simulink library "GTM_aerolib"  (R2023b)
settings: Solver=ode45  StartTime=0.0  StopTime=10.0  RelTol=1e-3
undefined symbols (not defined in the file or in its folder): Aero, DamageModels
libraries: simulink_need_slupdate x58, $bdroot x4, simulink x3
(part 1 of 2)
settings Model: Creator=cox  LastModifiedBy=suvo
settings SolverCC: AlgebraicLoopSolver=TrustRegion
settings DataIOCC: LimitDataPoints=on  SaveFormat=Array  SignalLoggingSaveFormat=ModelDataLogs  ReturnWorkspaceOutputs=off
settings OptimizationCC: BlockReduction=off  BooleanDataType=off  ExpressionDepthLimit=2147483647  LifeSpan=inf
settings DebuggingCC: SaveWithParameterizedLinksMsg=none  UnderspecifiedInitializationDetection=Classic  MergeDetectMultiDrivingBlocksExec=none  SignalResolutionControl=TryResolveAllWithWarning  FcnCallInpInsideContextMsg=warning  UnconnectedInputMsg=warning  UnconnectedOutputMsg=warning  UnconnectedLineMsg=warning  StateNameClashWarn=warning  SFUnexpectedBacktrackingDiag=warning  SFNoUnconditionalDefaultTransitionDiag=warning  SFExecutionAtInitializationDiag=none  ArithmeticOperatorsInVariantConditions=warning
settings HardwareCC: ProdBitPerPointer=32  ProdBitPerSizeT=32  ProdBitPerPtrDiffT=32  ProdLargestAtomicFloat=None  ProdIntDivRoundTo=Undefined  ProdEndianess=Unspecified  ProdWordSize=32  ProdHWDeviceType=32-bit Generic  TargetUnknown=on
settings ModelReferenceCC: PropagateSignalLabelsOutOfModel=off
settings SFSimCC: SimUseLocalCustomCode=off  CustomCodeUndefinedFunction=UseInterfaceOnly
settings RTWCC: RTWUseLocalCustomCode=off
settings CodeAppCC: StateflowObjectComments=on
settings GRTTargetCC: TargetLangStandard=C89/C90 (ANSI)  CombineOutputUpdateFcns=off  GRTInterface=on
settings ConfigComp: CovMetricSettings=dw  CovSaveCumulativeToWorkspaceVar=on  CovSaveSingleToWorkspaceVar=on

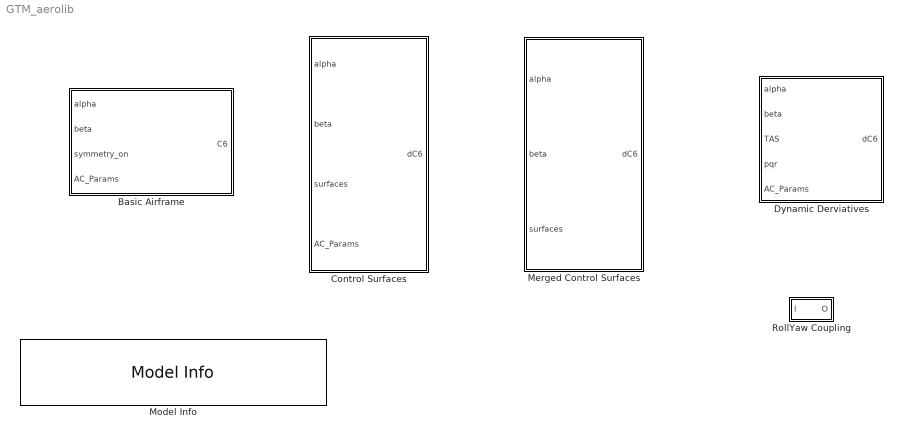
== system GTM_aerolib ==
  Basic Airframe : Subsystem
  Control Surfaces : Subsystem
  Dynamic Derviatives : Subsystem
  Merged Control Surfaces : Subsystem
  Model Info : simulink/Model-Wide Utilities/Model Info  Frame=on  DisplayStringWithTags=|  HorizontalTextAlignment=Center  LeftAlignmentValue=0.5
      | GTM AeroTables
      | Subversion Info: %<ModelVersion>
      | Last modified by %<LastModifiedBy> on %<LastModificationDate>
  RollYaw Coupling : Subsystem  mask{arm=-0.07}
      mask prompts: arm "Moment arm (nd)"
      mask help:
      | Approximates roll/yaw coupling of split longitudinal surface
      | deflections (spoilers, elevators, flaps) where the base aero data only
      | has CX, CZ, and Cm. Input should be a 6 element vector of the aero
      | coefficients [CZ CY CZ Cl Cm Cn].
      |
      | Cl = Cl_input + arm*CZ_input
      | Cn = Cn_input + arm*CX_input
      mask init:
      | Kc = eye(6);
      | 
      | Kc(4,3) = arm; % Cl = Cl + arm*CZ
      | Kc(6,1) = arm; % Cn = Cn + arm*CX

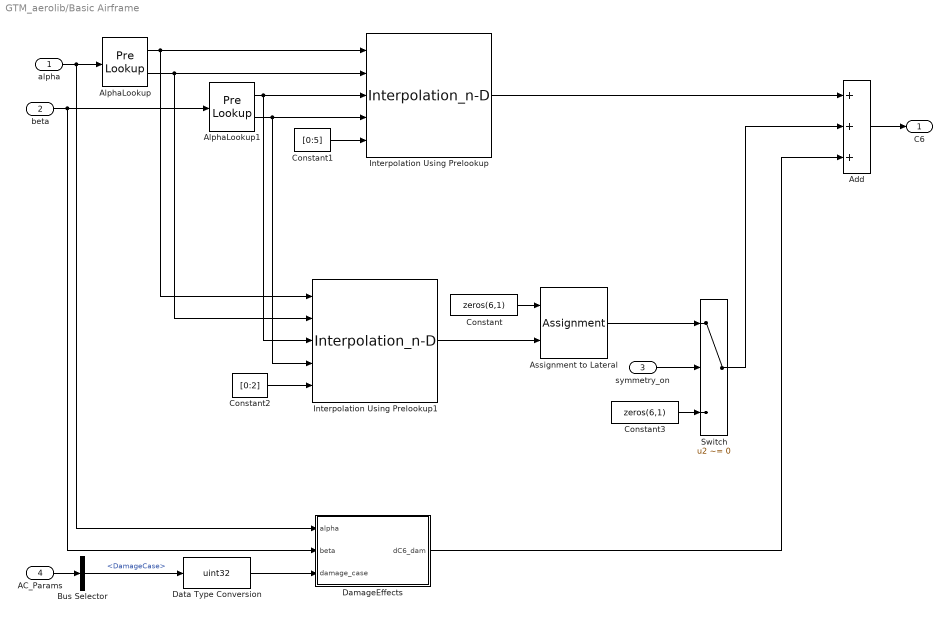
== system GTM_aerolib/Basic Airframe ==
  alpha : Inport
  beta : Inport  Port=2
  symmetry_on : Inport  Port=3
  AC_Params : Inport  Port=4
  Add : Sum  Inputs=+++
  AlphaLookup : PreLookup  BreakpointsData=Aero.C6_bas.alpha  IndexSearchMethod=Linear search  BeginIndexSearchUsingPreviousIndexResult=on  ExtrapMethod=Linear
  AlphaLookup1 : PreLookup  BreakpointsData=Aero.C6_bas.beta  IndexSearchMethod=Linear search  BeginIndexSearchUsingPreviousIndexResult=on  ExtrapMethod=Linear
  Assignment to Lateral : Assignment  IndexMode=Zero-based  IndexOptions=Index vector (dialog)  Indices=[1 3 5]  OutputSizes=[1 1]
  Bus Selector : BusSelector  OutputSignals=DamageCase
  Constant : Constant  Value=zeros(6,1)
  Constant1 : Constant  Value=[0:5]  OutDataTypeStr=uint32
  Constant2 : Constant  Value=[0:2]  OutDataTypeStr=uint32
  Constant3 : Constant  Value=zeros(6,1)
  DamageEffects : Subsystem
  Data Type Conversion : DataTypeConversion  OutDataTypeStr=uint32  RndMeth=Nearest  SaturateOnIntegerOverflow=off
  Interpolation Using Prelookup : Interpolation_n-D  NumberOfTableDimensions=3  Table=Aero.C6_bas.data  NumSelectionDims=1
      settings: InputPortMap=u0,u1,u2,u3,u4
  Interpolation Using Prelookup1 : Interpolation_n-D  NumberOfTableDimensions=3  Table=Aero.dC3_sym.data  NumSelectionDims=1
      settings: InputPortMap=u0,u1,u2,u3,u4
  Switch : Switch  Criteria=u2 ~= 0  SaturateOnIntegerOverflow=off  InputSameDT=off
  C6 : Outport
  wires:
  Interpolation Using Prelookup/1 -> Add/1
  Constant/1 -> Assignment to Lateral/1
  Interpolation Using Prelookup1/1 -> Assignment to Lateral/2
  Constant3/1 -> Switch/3
  Assignment to Lateral/1 -> Switch/1
  symmetry_on/1 -> Switch/2
  Add/1 -> C6/1
  Switch/1 -> Add/2
  alpha/1 -> DamageEffects/1(alpha), AlphaLookup/1
  beta/1 -> DamageEffects/2(beta), AlphaLookup1/1
  DamageEffects/1(dC6_dam) -> Add/3
  AC_Params/1 -> Bus Selector/1
  Bus Selector/1 -> Data Type Conversion/1  "<DamageCase>"
  AlphaLookup/1 -> Interpolation Using Prelookup/1, Interpolation Using Prelookup1/1
  AlphaLookup/2 -> Interpolation Using Prelookup/2, Interpolation Using Prelookup1/2
  AlphaLookup1/1 -> Interpolation Using Prelookup/3, Interpolation Using Prelookup1/3
  AlphaLookup1/2 -> Interpolation Using Prelookup/4, Interpolation Using Prelookup1/4
  Constant1/1 -> Interpolation Using Prelookup/5
  Constant2/1 -> Interpolation Using Prelookup1/5
  Data Type Conversion/1 -> DamageEffects/3(damage_case)

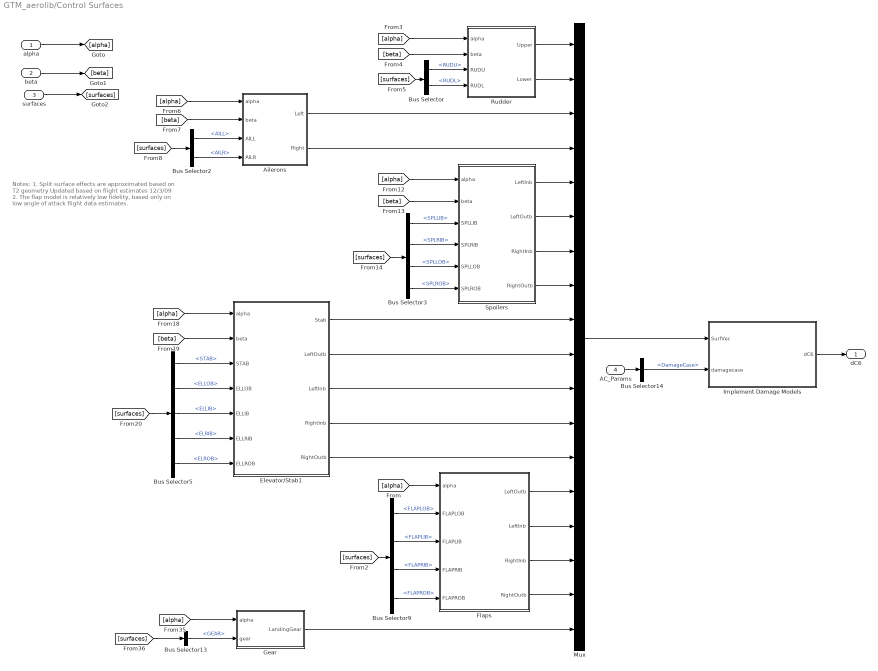
== system GTM_aerolib/Control Surfaces ==
  note: Notes:
      | 1. Split surface effects are approximated
      | based on T2 geometry
      | Updated based on flight estimates 12/3/09
      |
      | 2. The flap model is relatively low fidelity, based
      | only on low angle of attack flight data estimates.
  alpha : Inport
  beta : Inport  Port=2  PortDimensions=1
  surfaces : Inport  Port=3
  AC_Params : Inport  Port=4
  Ailerons : Subsystem
  Bus Selector : BusSelector  OutputSignals=RUDU,RUDL
  Bus Selector13 : BusSelector  OutputSignals=GEAR
  Bus Selector14 : BusSelector  OutputSignals=DamageCase
  Bus Selector2 : BusSelector  OutputSignals=AILL,AILR
  Bus Selector3 : BusSelector  OutputSignals=SPLLIB,SPLRIB,SPLLOB,SPLROB
  Bus Selector5 : BusSelector  OutputSignals=STAB,ELLOB,ELLIB,ELRIB,ELROB
  Bus Selector9 : BusSelector  OutputSignals=FLAPLOB,FLAPLIB,FLAPRIB,FLAPROB
  Elevator/Stab1 : Subsystem
  Flaps : Subsystem
  Gear : Subsystem
  Implement Damage Models : Subsystem  mask{DamageModels=DamageModels}
      mask prompts: DamageModels "Cell Array of Damage Models"
      mask help: Implements Damage Models as gain and bias effects on selected surfaces.
      mask init:
      | SurfList={...
      |     'RUDU','RUDL',...
      |     'AILL','AILR',...
      |     'SPLLIB','SPLRIB','SPLLOB','SPLROB',...
      |     'STAB',...
      |     'ELLOB','ELLIB','ELRIB','ELROB',...
      |     'FLAPLOB','FALPLIB','FLAPRIB','FLAPROB',...
      |     'GEAR'
      |     };
      | 
      | Ncases=length(DamageModels);
      | Nsurfs=length(SurfList);
      | SurfGain=ones(Ncases,Nsurfs,6);   %Nominally unity gain, zero bias
      | 
      | %If damage case includes gain/bias on a surface adjust nominal values
      | % First damage case is "no damage".
      | for i=1:Ncases,
      |  for j=1:Nsurfs,
      |     if isfield(DamageModels{i},SurfList{j}),
      |         SurfGain(i,j,:)=DamageModels{i}.(SurfList{j}).gain*ones(1,6);
      |     end
      |  end
      | end
  Mux : Mux  Inputs=18
  Rudder : Subsystem
  Spoilers : Subsystem
  dC6 : Outport
  wires:
  Bus Selector13/1 -> Gear/2(gear)  "<GEAR>"
  [alpha] -> Gear/1(alpha)
  [surfaces] -> Bus Selector13/1
  [alpha] -> Flaps/1(alpha)
  [surfaces] -> Bus Selector9/1
  Bus Selector5/2 -> Elevator/Stab1/4(ELLOB)  "<ELLOB>"
  Bus Selector5/1 -> Elevator/Stab1/3(STAB)  "<STAB>"
  [alpha] -> Elevator/Stab1/1(alpha)
  [surfaces] -> Bus Selector5/1
  [beta] -> Elevator/Stab1/2(beta)
  Bus Selector3/2 -> Spoilers/4(SPLRIB)  "<SPLRIB>"
  Bus Selector3/1 -> Spoilers/3(SPLLIB)  "<SPLLIB>"
  [surfaces] -> Bus Selector3/1
  [beta] -> Spoilers/2(beta)
  [alpha] -> Spoilers/1(alpha)
  Bus Selector2/2 -> Ailerons/4(AILR)  "<AILR>"
  Bus Selector2/1 -> Ailerons/3(AILL)  "<AILL>"
  [surfaces] -> Bus Selector2/1
  [beta] -> Ailerons/2(beta)
  [alpha] -> Ailerons/1(alpha)
  Bus Selector/2 -> Rudder/4(RUDL)  "<RUDL>"
  Bus Selector/1 -> Rudder/3(RUDU)  "<RUDU>"
  [surfaces] -> Bus Selector/1
  [beta] -> Rudder/2(beta)
  [alpha] -> Rudder/1(alpha)
  surfaces/1 -> [surfaces]
  beta/1 -> [beta]
  alpha/1 -> [alpha]
  AC_Params/1 -> Bus Selector14/1
  Bus Selector3/3 -> Spoilers/5(SPLLOB)  "<SPLLOB>"
  Bus Selector3/4 -> Spoilers/6(SPLROB)  "<SPLROB>"
  Bus Selector5/3 -> Elevator/Stab1/5(ELLIB)  "<ELLIB>"
  Bus Selector5/4 -> Elevator/Stab1/6(ELLRIB)  "<ELRIB>"
  Bus Selector5/5 -> Elevator/Stab1/7(ELLROB)  "<ELROB>"
  Rudder/1(Upper) -> Mux/1
  Rudder/2(Lower) -> Mux/2
  Ailerons/1(Left) -> Mux/3
  Ailerons/2(Right) -> Mux/4
  Spoilers/1(LeftInb) -> Mux/5
  Spoilers/2(LeftOutb) -> Mux/6
  Spoilers/3(RightInb) -> Mux/7
  Spoilers/4(RightOutb) -> Mux/8
  Elevator/Stab1/1(Stab) -> Mux/9
  Elevator/Stab1/2(LeftOutb) -> Mux/10
  Elevator/Stab1/3(LeftInb) -> Mux/11
  Elevator/Stab1/4(RightInb) -> Mux/12
  Elevator/Stab1/5(RightOutb) -> Mux/13
  Gear/1(LandingGear) -> Mux/18
  Flaps/1(LeftOutb) -> Mux/14
  Flaps/2(LeftInb) -> Mux/15
  Flaps/3(RightInb) -> Mux/16
  Flaps/4(RightOutb) -> Mux/17
  Bus Selector14/1 -> Implement Damage Models/2(damagecase)  "<DamageCase>"
  Mux/1 -> Implement Damage Models/1(SurfVec)
  Implement Damage Models/1(dC6) -> dC6/1
  Bus Selector9/1 -> Flaps/2(FLAPLOB)  "<FLAPLOB>"
  Bus Selector9/2 -> Flaps/3(FLAPLIB)  "<FLAPLIB>"
  Bus Selector9/3 -> Flaps/4(FLAPRIB)  "<FLAPRIB>"
  Bus Selector9/4 -> Flaps/5(FLAPROB)  "<FLAPROB>"

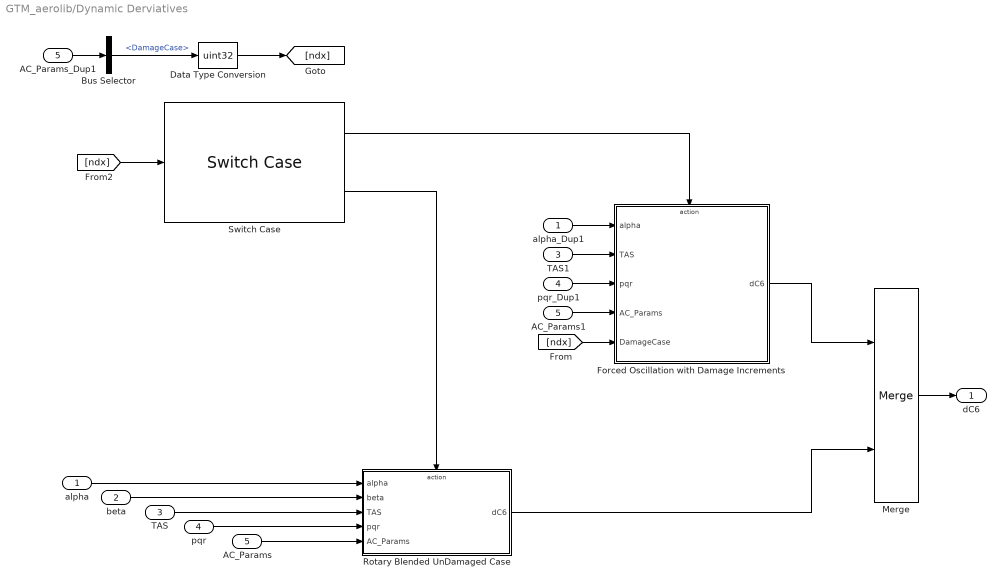
== system GTM_aerolib/Dynamic Derviatives ==
  alpha : Inport
  beta : Inport  Port=2
  TAS : Inport  Port=3
  pqr : Inport  Port=4
  AC_Params : Inport  Port=5
  AC_Params1 : InportShadow  Port=5
  AC_Params_Dup1 : InportShadow  Port=5
  Bus Selector : BusSelector  OutputSignals=DamageCase
  Data Type Conversion : DataTypeConversion  OutDataTypeStr=uint32  RndMeth=Nearest  SaturateOnIntegerOverflow=off
  Forced Oscillation with Damage Increments : Subsystem
  Merge : Merge  InitialOutput=zeros(6,1)
  Rotary Blended UnDamaged Case : Subsystem
  Switch Case : SwitchCase  CaseConditions={[1,2,3,4,5,6]}
  TAS1 : InportShadow  Port=3
  alpha_Dup1 : InportShadow
  pqr_Dup1 : InportShadow  Port=4
  dC6 : Outport
  wires:
  alpha/1 -> Rotary Blended UnDamaged Case/1(alpha)
  beta/1 -> Rotary Blended UnDamaged Case/2(beta)
  TAS/1 -> Rotary Blended UnDamaged Case/3(TAS)
  pqr/1 -> Rotary Blended UnDamaged Case/4(pqr)
  AC_Params/1 -> Rotary Blended UnDamaged Case/5(AC_Params)
  Merge/1 -> dC6/1
  Switch Case/1 -> Forced Oscillation with Damage Increments/Action
  Switch Case/2 -> Rotary Blended UnDamaged Case/Action
  Rotary Blended UnDamaged Case/1(dC6) -> Merge/2
  Bus Selector/1 -> Data Type Conversion/1  "<DamageCase>"
  AC_Params_Dup1/1 -> Bus Selector/1
  Data Type Conversion/1 -> [ndx]
  [ndx] -> Switch Case/1
  alpha_Dup1/1 -> Forced Oscillation with Damage Increments/1(alpha)
  TAS1/1 -> Forced Oscillation with Damage Increments/2(TAS)
  pqr_Dup1/1 -> Forced Oscillation with Damage Increments/3(pqr)
  AC_Params1/1 -> Forced Oscillation with Damage Increments/4(AC_Params)
  [ndx] -> Forced Oscillation with Damage Increments/5(DamageCase)
  Forced Oscillation with Damage Increments/1(dC6) -> Merge/1

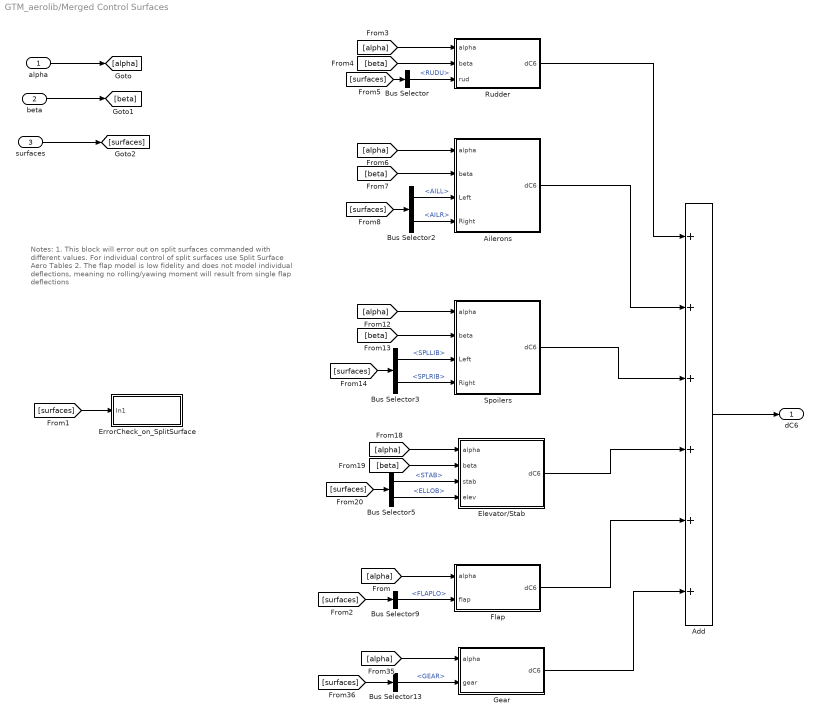
== system GTM_aerolib/Merged Control Surfaces ==
  note: Notes:
      | 1. This block will error out on split surfaces commanded
      | with different values.  For individual control of split surfaces
      | use Split Surface Aero Tables
      |
      | 2. The flap model is low fidelity and does
      | not model individual deflections, meaning
      | no rolling/yawing moment will result
      | from single flap deflections
  alpha : Inport
  beta : Inport  Port=2  PortDimensions=1
  surfaces : Inport  Port=3
  Add : Sum  Inputs=++++++
  Ailerons : Subsystem
  Bus Selector : BusSelector  OutputSignals=RUDU
  Bus Selector13 : BusSelector  OutputSignals=GEAR
  Bus Selector2 : BusSelector  OutputSignals=AILL,AILR
  Bus Selector3 : BusSelector  OutputSignals=SPLLIB,SPLRIB
  Bus Selector5 : BusSelector  OutputSignals=STAB,ELLOB
  Bus Selector9 : BusSelector  OutputSignals=FLAPLO
  Elevator/Stab : Subsystem
  ErrorCheck_on_SplitSurface : Subsystem
  Flap : Subsystem
  Gear : Subsystem
  Rudder : Subsystem
  Spoilers : Subsystem
  dC6 : Outport
  wires:
  Add/1 -> dC6/1
  alpha/1 -> [alpha]
  beta/1 -> [beta]
  surfaces/1 -> [surfaces]
  [alpha] -> Rudder/1(alpha)
  [beta] -> Rudder/2(beta)
  [surfaces] -> Bus Selector/1
  Bus Selector/1 -> Rudder/3(rud)  "<RUDU>"
  [alpha] -> Ailerons/1(alpha)
  [beta] -> Ailerons/2(beta)
  [surfaces] -> Bus Selector2/1
  Bus Selector2/1 -> Ailerons/3(Left)  "<AILL>"
  Bus Selector2/2 -> Ailerons/4(Right)  "<AILR>"
  [alpha] -> Spoilers/1(alpha)
  [beta] -> Spoilers/2(beta)
  [surfaces] -> Bus Selector3/1
  Bus Selector3/1 -> Spoilers/3(Left)  "<SPLLIB>"
  Bus Selector3/2 -> Spoilers/4(Right)  "<SPLRIB>"
  [beta] -> Elevator/Stab/2(beta)
  [surfaces] -> Bus Selector5/1
  [alpha] -> Elevator/Stab/1(alpha)
  Bus Selector5/1 -> Elevator/Stab/3(stab)  "<STAB>"
  Bus Selector5/2 -> Elevator/Stab/4(elev)  "<ELLOB>"
  [surfaces] -> Bus Selector9/1
  [alpha] -> Flap/1(alpha)
  Bus Selector9/1 -> Flap/2(flap)  "<FLAPLO>"
  [surfaces] -> Bus Selector13/1
  [alpha] -> Gear/1(alpha)
  Bus Selector13/1 -> Gear/2(gear)  "<GEAR>"
  Rudder/1(dC6) -> Add/1
  Ailerons/1(dC6) -> Add/2
  Spoilers/1(dC6) -> Add/3
  Elevator/Stab/1(dC6) -> Add/4
  Flap/1(dC6) -> Add/5
  Gear/1(dC6) -> Add/6
  [surfaces] -> ErrorCheck_on_SplitSurface/1(In1)

== system GTM_aerolib/RollYaw Coupling ==
  I : Inport
  Gain : Gain  Gain=Kc  Multiplication=Matrix(K*u)
  O : Outport
  wires:
  I/1 -> Gain/1
  Gain/1 -> O/1

== system GTM_aerolib/Basic Airframe/DamageEffects ==
  alpha : Inport
  beta : Inport  Port=2
  damage_case : Inport  Port=3
  Merge : Merge  InitialOutput=zeros(6,1)
  Switch Case : SwitchCase  CaseConditions={[1,2,3,4,5,6]}
  Switch Case Action Subsystem : Subsystem  TreatAsAtomicUnit=on
  Switch Case Action Subsystem2 : Subsystem  TreatAsAtomicUnit=on
  damage_case_DUP : InportShadow  Port=3
  dC6_dam : Outport
  wires:
  Switch Case/2 -> Switch Case Action Subsystem2/Action
  Switch Case Action Subsystem2/1(Zeros) -> Merge/2
  alpha/1 -> Switch Case Action Subsystem/1(alpha)
  beta/1 -> Switch Case Action Subsystem/2(beta)
  Merge/1 -> dC6_dam/1
  damage_case/1 -> Switch Case/1
  Switch Case/1 -> Switch Case Action Subsystem/Action
  Switch Case Action Subsystem/1(dC6_dam) -> Merge/1
  damage_case_DUP/1 -> Switch Case Action Subsystem/3(damage_case)

== system GTM_aerolib/Control Surfaces/Ailerons ==
  alpha : Inport
  beta : Inport  Port=2
  AILL : Inport  Port=3
  AILR : Inport  Port=4
  Constant1 : Constant  Value=[0:5]  OutDataTypeStr=uint32
  Constant3 : Constant  Value=[0:5]  OutDataTypeStr=uint32
  Gain2 : Gain  Gain=-1
  Interpolation Using Prelookup : Interpolation_n-D  NumberOfTableDimensions=4  Table=Aero.dC6_ail.data  NumSelectionDims=1
      settings: InputPortMap=u0,u1,u2,u3,u4,u5,u6
  Interpolation Using Prelookup1 : Interpolation_n-D  NumberOfTableDimensions=4  Table=Aero.dC6_ail.data  NumSelectionDims=1
      settings: InputPortMap=u0,u1,u2,u3,u4,u5,u6
  Negate Lateral : Gain  Gain=[1 -1 1 -1 1 -1]
  Prelookup1 : PreLookup  BreakpointsData=Aero.dC6_ail.alpha  IndexSearchMethod=Linear search  BeginIndexSearchUsingPreviousIndexResult=on  ExtrapMethod=Linear
  Prelookup2 : PreLookup  BreakpointsData=Aero.dC6_ail.beta  IndexSearchMethod=Linear search  BeginIndexSearchUsingPreviousIndexResult=on  ExtrapMethod=Linear
  Prelookup3 : PreLookup  BreakpointsData=Aero.dC6_ail.ail  IndexSearchMethod=Linear search  BeginIndexSearchUsingPreviousIndexResult=on  ExtrapMethod=Linear
  Prelookup4 : PreLookup  BreakpointsData=Aero.dC6_ail.beta  IndexSearchMethod=Linear search  BeginIndexSearchUsingPreviousIndexResult=on  ExtrapMethod=Linear
  Prelookup5 : PreLookup  BreakpointsData=Aero.dC6_ail.ail  IndexSearchMethod=Linear search  BeginIndexSearchUsingPreviousIndexResult=on  ExtrapMethod=Linear
  Left : Outport
  Right : Outport  Port=2
  wires:
  Gain2/1 -> Prelookup2/1
  Negate Lateral/1 -> Left/1
  Interpolation Using Prelookup1/1 -> Right/1
  AILR/1 -> Prelookup5/1
  beta/1 -> Gain2/1, Prelookup4/1
  alpha/1 -> Prelookup1/1
  AILL/1 -> Prelookup3/1
  Prelookup1/1 -> Interpolation Using Prelookup/1, Interpolation Using Prelookup1/1
  Prelookup1/2 -> Interpolation Using Prelookup/2, Interpolation Using Prelookup1/2
  Prelookup2/1 -> Interpolation Using Prelookup/3
  Prelookup2/2 -> Interpolation Using Prelookup/4
  Prelookup3/1 -> Interpolation Using Prelookup/5
  Prelookup3/2 -> Interpolation Using Prelookup/6
  Constant3/1 -> Interpolation Using Prelookup/7
  Prelookup4/1 -> Interpolation Using Prelookup1/3
  Prelookup4/2 -> Interpolation Using Prelookup1/4
  Prelookup5/1 -> Interpolation Using Prelookup1/5
  Prelookup5/2 -> Interpolation Using Prelookup1/6
  Constant1/1 -> Interpolation Using Prelookup1/7
  Interpolation Using Prelookup/1 -> Negate Lateral/1

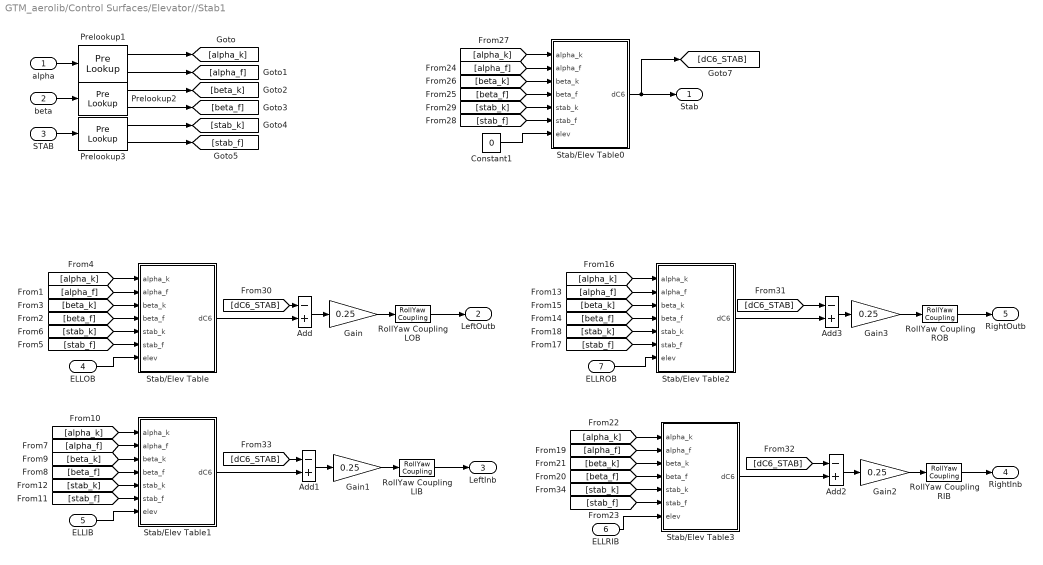
== system GTM_aerolib/Control Surfaces/Elevator//Stab1 ==
  alpha : Inport
  beta : Inport  Port=2
  STAB : Inport  Port=3
  ELLOB : Inport  Port=4
  ELLIB : Inport  Port=5
  ELLRIB : Inport  Port=6
  ELLROB : Inport  Port=7
  Add{,1..3} (4 alike) : Sum  Inputs=-+
  Constant1 : Constant  Value=0
  Gain{,1..3} (4 alike) : Gain  Gain=0.25
  Prelookup1 : PreLookup  BreakpointsData=Aero.dC3_ele.alpha  IndexSearchMethod=Linear search  BeginIndexSearchUsingPreviousIndexResult=on  ExtrapMethod=Linear
  Prelookup2 : PreLookup  BreakpointsData=Aero.dC3_ele.beta  IndexSearchMethod=Linear search  BeginIndexSearchUsingPreviousIndexResult=on  ExtrapMethod=Linear
  Prelookup3 : PreLookup  BreakpointsData=Aero.dC3_ele.stab  IndexSearchMethod=Linear search  BeginIndexSearchUsingPreviousIndexResult=on  ExtrapMethod=Linear
  RollYaw Coupling LIB : $bdroot/RollYaw Coupling  SystemSampleTime=-1  arm=-0.03
  RollYaw Coupling LOB : $bdroot/RollYaw Coupling  SystemSampleTime=-1  arm=-0.07
  RollYaw Coupling RIB : $bdroot/RollYaw Coupling  SystemSampleTime=-1  arm=0.03
  RollYaw Coupling ROB : $bdroot/RollYaw Coupling  SystemSampleTime=-1  arm=0.07
  Stab/Elev Table : Subsystem
  Stab/Elev Table0 : Subsystem
  Stab/Elev Table1 : Subsystem
  Stab/Elev Table2 : Subsystem
  Stab/Elev Table3 : Subsystem
  Stab : Outport
  LeftOutb : Outport  Port=2
  LeftInb : Outport  Port=3
  RightInb : Outport  Port=4
  RightOutb : Outport  Port=5
  wires:
  alpha/1 -> Prelookup1/1
  beta/1 -> Prelookup2/1
  STAB/1 -> Prelookup3/1
  Prelookup1/1 -> [alpha_k]
  Prelookup1/2 -> [alpha_f]
  Prelookup2/1 -> [beta_k]
  Prelookup2/2 -> [beta_f]
  Prelookup3/1 -> [stab_k]
  Prelookup3/2 -> [stab_f]
  Gain/1 -> RollYaw Coupling LOB/1
  Gain1/1 -> RollYaw Coupling LIB/1
  Gain2/1 -> RollYaw Coupling RIB/1
  Gain3/1 -> RollYaw Coupling ROB/1
  Add/1 -> Gain/1
  Add1/1 -> Gain1/1
  Add2/1 -> Gain2/1
  Add3/1 -> Gain3/1
  [alpha_k] -> Stab/Elev Table/1(alpha_k)
  [alpha_f] -> Stab/Elev Table/2(alpha_f)
  [beta_k] -> Stab/Elev Table/3(beta_k)
  [beta_f] -> Stab/Elev Table/4(beta_f)
  [stab_k] -> Stab/Elev Table/5(stab_k)
  [stab_f] -> Stab/Elev Table/6(stab_f)
  ELLOB/1 -> Stab/Elev Table/7(elev)
  [alpha_k] -> Stab/Elev Table1/1(alpha_k)
  [alpha_f] -> Stab/Elev Table1/2(alpha_f)
  [beta_k] -> Stab/Elev Table1/3(beta_k)
  [beta_f] -> Stab/Elev Table1/4(beta_f)
  [stab_k] -> Stab/Elev Table1/5(stab_k)
  [stab_f] -> Stab/Elev Table1/6(stab_f)
  ELLIB/1 -> Stab/Elev Table1/7(elev)
  [alpha_k] -> Stab/Elev Table2/1(alpha_k)
  [alpha_f] -> Stab/Elev Table2/2(alpha_f)
  [beta_k] -> Stab/Elev Table2/3(beta_k)
  [beta_f] -> Stab/Elev Table2/4(beta_f)
  [stab_k] -> Stab/Elev Table2/5(stab_k)
  [stab_f] -> Stab/Elev Table2/6(stab_f)
  ELLROB/1 -> Stab/Elev Table2/7(elev)
  [alpha_k] -> Stab/Elev Table3/1(alpha_k)
  [alpha_f] -> Stab/Elev Table3/2(alpha_f)
  [beta_k] -> Stab/Elev Table3/3(beta_k)
  [beta_f] -> Stab/Elev Table3/4(beta_f)
  [stab_k] -> Stab/Elev Table3/5(stab_k)
  [stab_f] -> Stab/Elev Table3/6(stab_f)
  ELLRIB/1 -> Stab/Elev Table3/7(elev)
  Stab/Elev Table/1(dC6) -> Add/2
  [dC6_STAB] -> Add/1
  [alpha_k] -> Stab/Elev Table0/1(alpha_k)
  [alpha_f] -> Stab/Elev Table0/2(alpha_f)
  [beta_k] -> Stab/Elev Table0/3(beta_k)
  [beta_f] -> Stab/Elev Table0/4(beta_f)
  [stab_k] -> Stab/Elev Table0/5(stab_k)
  [stab_f] -> Stab/Elev Table0/6(stab_f)
  Constant1/1 -> Stab/Elev Table0/7(elev)
  Stab/Elev Table1/1(dC6) -> Add1/2
  Stab/Elev Table2/1(dC6) -> Add3/2
  [dC6_STAB] -> Add3/1
  [dC6_STAB] -> Add2/1
  Stab/Elev Table3/1(dC6) -> Add2/2
  [dC6_STAB] -> Add1/1
  Stab/Elev Table0/1(dC6) -> Stab/1, [dC6_STAB]
  RollYaw Coupling LOB/1 -> LeftOutb/1
  RollYaw Coupling LIB/1 -> LeftInb/1
  RollYaw Coupling ROB/1 -> RightOutb/1
  RollYaw Coupling RIB/1 -> RightInb/1

== system GTM_aerolib/Control Surfaces/Flaps ==
  alpha : Inport
  FLAPLOB : Inport  Port=2
  FLAPLIB : Inport  Port=3
  FLAPRIB : Inport  Port=4
  FLAPROB : Inport  Port=5
  Gain : Gain  Gain=Aero.flaps.flaplob
  Gain1 : Gain  Gain=Aero.flaps.flaplib
  Gain2 : Gain  Gain=Aero.flaps.flaprib
  Gain3 : Gain  Gain=Aero.flaps.flaprob
  Terminator : Terminator
  LeftOutb : Outport
  LeftInb : Outport  Port=2
  RightInb : Outport  Port=3
  RightOutb : Outport  Port=4
  wires:
  alpha/1 -> Terminator/1
  FLAPLOB/1 -> Gain/1
  FLAPLIB/1 -> Gain1/1
  FLAPRIB/1 -> Gain2/1
  FLAPROB/1 -> Gain3/1
  Gain/1 -> LeftOutb/1
  Gain1/1 -> LeftInb/1
  Gain2/1 -> RightInb/1
  Gain3/1 -> RightOutb/1

== system GTM_aerolib/Control Surfaces/Gear ==
  alpha : Inport
  gear : Inport  Port=2
  Assignment to Longitudinal : Assignment  IndexMode=Zero-based  IndexOptions=Index vector (dialog)  Indices=[0 2 4]  OutputSizes=[1 1]
  Compare To Zero : simulink/Logic and Bit Operations/Compare To Zero  SystemSampleTime=-1  relop=~=  LogicOutDataTypeMode=uint8  ZeroCross=off
  Constant : Constant  Value=zeros(6,1)
  Constant2 : Constant  Value=[0:2]  OutDataTypeStr=uint32
  Data Type Conversion2 : DataTypeConversion  OutDataTypeStr=uint32  SaturateOnIntegerOverflow=off  RndMeth=Floor
  PreLookup Index Search1 : simulink_need_slupdate/PreLookup Index Search  bpData=Aero.dC3_lgr.alpha  searchMode=Binary Search  cacheBpFlag=on  outputFlag=off  IndexDataType=uint32  extrapMode=Linear Extrapolation  rangeErrorMode=None
  TableLookup : simulink_need_slupdate/Interpolation (n-D) using PreLookup  numDimsPopupSelect=3  explicitNumDims=2  table=Aero.dC3_lgr.data  interpMethod=Linear  extrapMethod=Linear  rangeErrorMode=None  NumSelectionDims=2
  LandingGear : Outport
  wires:
  Data Type Conversion2/1 -> TableLookup/2
  Assignment to Longitudinal/1 -> LandingGear/1
  Constant/1 -> Assignment to Longitudinal/1
  TableLookup/1 -> Assignment to Longitudinal/2
  Constant2/1 -> TableLookup/3
  PreLookup Index Search1/1 -> TableLookup/1
  alpha/1 -> PreLookup Index Search1/1
  Compare To Zero/1 -> Data Type Conversion2/1
  gear/1 -> Compare To Zero/1

== system GTM_aerolib/Control Surfaces/Implement Damage Models ==
  SurfVec : Inport
  damagecase : Inport  Port=2
  Implement Damage Models : MATLAB Function  TreatAsAtomicUnit=on
  Reshape : Reshape
  dC6 : Outport
  wires:
  SurfVec/1 -> Implement Damage Models/1(SurfVec)
  Implement Damage Models/1(dC6) -> Reshape/1
  damagecase/1 -> Implement Damage Models/2(DamageCase)
  Reshape/1 -> dC6/1

== system GTM_aerolib/Control Surfaces/Rudder ==
  alpha : Inport
  beta : Inport  Port=2
  RUDU : Inport  Port=3
  RUDL : Inport  Port=4
  Gains : Subsystem  mask{gains=[0.5  0.5  0.5  0.67  0.67  0.5]}
      mask prompts: gains "Mask Parameter 1:"
      mask help: Gains for each aerodynamic coefficient.
      mask Display: disp(['[' num2str(gains) ']'])
  Gains1 : Subsystem  mask{gains=[0.5  0.5  0.5  0.33  0.33  0.5]}
      mask prompts: gains "Mask Parameter 1:"
      mask help: Gains for each aerodynamic coefficient.
      mask Display: disp(['[' num2str(gains) ']'])
  Lower Rudder : Subsystem
  Upper Rudder : Subsystem
  Upper : Outport
  Lower : Outport  Port=2
  wires:
  Lower Rudder/1(dC6) -> Gains1/1(dC6_in)
  Upper Rudder/1(dC6) -> Gains/1(dC6_in)
  alpha/1 -> Upper Rudder/1(alpha), Lower Rudder/1(alpha)
  Gains/1(dC6) -> Upper/1
  beta/1 -> Upper Rudder/2(beta), Lower Rudder/2(beta)
  RUDU/1 -> Upper Rudder/3(rud)
  Gains1/1(dC6) -> Lower/1
  RUDL/1 -> Lower Rudder/3(rud)

== system GTM_aerolib/Control Surfaces/Spoilers ==
  alpha : Inport
  beta : Inport  Port=2
  SPLLIB : Inport  Port=3
  SPLRIB : Inport  Port=4
  SPLLOB : Inport  Port=5
  SPLROB : Inport  Port=6
  Gains1 : Subsystem  mask{gains=|}
      mask gains=|
      | [0.45	0.45	0.45	0.26	0.45	0.26
      | ]
      mask prompts: gains "Mask Parameter 1:"
      mask help: Gains for each aerodynamic coefficient.
      mask Display: disp(['[' num2str(gains) ']'])
  Gains2 : Subsystem  mask{gains=|}
      mask gains=|
      | [0.45	0.45	0.45	0.26	0.45	0.26
      | ]
      mask prompts: gains "Mask Parameter 1:"
      mask help: Gains for each aerodynamic coefficient.
      mask Display: disp(['[' num2str(gains) ']'])
  Gains3 : Subsystem  mask{gains=|}
      mask gains=|
      | [0.55	0.55	0.55	0.74	0.55	0.74
      | ]
      mask prompts: gains "Mask Parameter 1:"
      mask help: Gains for each aerodynamic coefficient.
      mask Display: disp(['[' num2str(gains) ']'])
  Gains4 : Subsystem  mask{gains=|}
      mask gains=|
      | [0.55	0.55	0.55	0.74	0.55	0.74
      | ]
      mask prompts: gains "Mask Parameter 1:"
      mask help: Gains for each aerodynamic coefficient.
      mask Display: disp(['[' num2str(gains) ']'])
  InboardSpoilers : Subsystem
  OutboardSpoilers : Subsystem
  LeftInb : Outport
  LeftOutb : Outport  Port=2
  RightInb : Outport  Port=3
  RightOutb : Outport  Port=4
  wires:
  InboardSpoilers/1(Left) -> Gains2/1(dC6_in)
  OutboardSpoilers/1(Left) -> Gains3/1(dC6_in)
  alpha/1 -> InboardSpoilers/1(alpha), OutboardSpoilers/1(alpha)
  beta/1 -> InboardSpoilers/2(beta), OutboardSpoilers/2(beta)
  Gains2/1(dC6) -> LeftInb/1
  SPLLIB/1 -> InboardSpoilers/3(SPLLIB)
  SPLRIB/1 -> InboardSpoilers/4(SPLRIB)
  Gains3/1(dC6) -> LeftOutb/1
  SPLLOB/1 -> OutboardSpoilers/3(SPLLIB)
  SPLROB/1 -> OutboardSpoilers/4(SPLRIB)
  InboardSpoilers/2(Right) -> Gains1/1(dC6_in)
  Gains1/1(dC6) -> RightInb/1
  OutboardSpoilers/2(Right) -> Gains4/1(dC6_in)
  Gains4/1(dC6) -> RightOutb/1

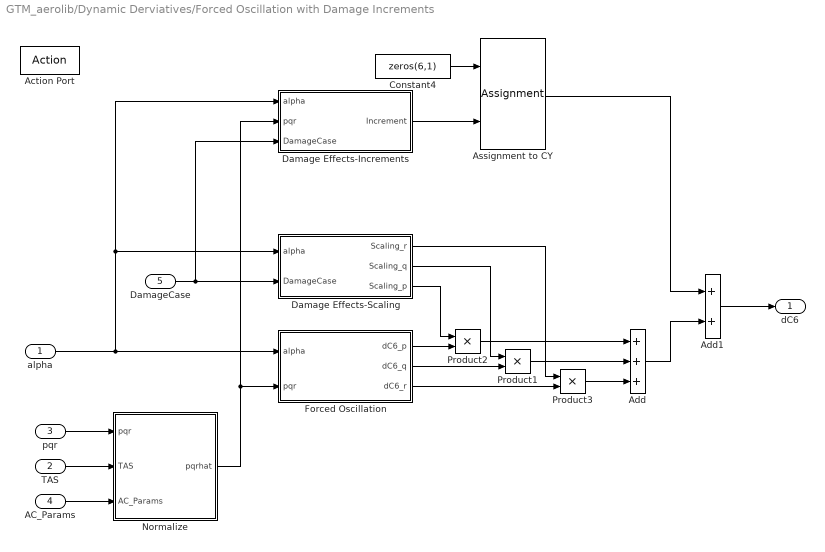
== system GTM_aerolib/Dynamic Derviatives/Forced Oscillation with Damage Increments ==
  alpha : Inport
  TAS : Inport  Port=2
  pqr : Inport  Port=3
  AC_Params : Inport  Port=4
  DamageCase : Inport  Port=5
  Action Port : ActionPort
  Add : Sum  Inputs=+++
  Add1 : Sum
  Assignment to CY : Assignment  IndexMode=Zero-based  IndexOptions=Index vector (dialog)  Indices=1  OutputSizes=[1 1]
  Constant4 : Constant  Value=zeros(6,1)
  Damage Effects-Increments : Subsystem
  Damage Effects-Scaling : Subsystem
  Forced Oscillation : Subsystem
  Normalize : Subsystem
  Product1 : Product  RndMeth=Zero
  Product2 : Product  RndMeth=Zero
  Product3 : Product  RndMeth=Zero
  dC6 : Outport
  wires:
  alpha/1 -> Forced Oscillation/1(alpha), Damage Effects-Scaling/1(alpha), Damage Effects-Increments/1(alpha)
  DamageCase/1 -> Damage Effects-Scaling/2(DamageCase), Damage Effects-Increments/3(DamageCase)
  Damage Effects-Scaling/1(Scaling_r) -> Product3/1
  Damage Effects-Scaling/2(Scaling_q) -> Product1/1
  Damage Effects-Scaling/3(Scaling_p) -> Product2/1
  Damage Effects-Increments/1(Increment) -> Assignment to CY/2
  Constant4/1 -> Assignment to CY/1
  Add1/1 -> dC6/1
  pqr/1 -> Normalize/1(pqr)
  TAS/1 -> Normalize/2(TAS)
  AC_Params/1 -> Normalize/3(AC_Params)
  Normalize/1(pqrhat) -> Forced Oscillation/2(pqr), Damage Effects-Increments/2(pqr)
  Forced Oscillation/1(dC6_p) -> Product2/2
  Forced Oscillation/2(dC6_q) -> Product1/2
  Forced Oscillation/3(dC6_r) -> Product3/2
  Product3/1 -> Add/3
  Product1/1 -> Add/2
  Product2/1 -> Add/1
  Add/1 -> Add1/2
  Assignment to CY/1 -> Add1/1

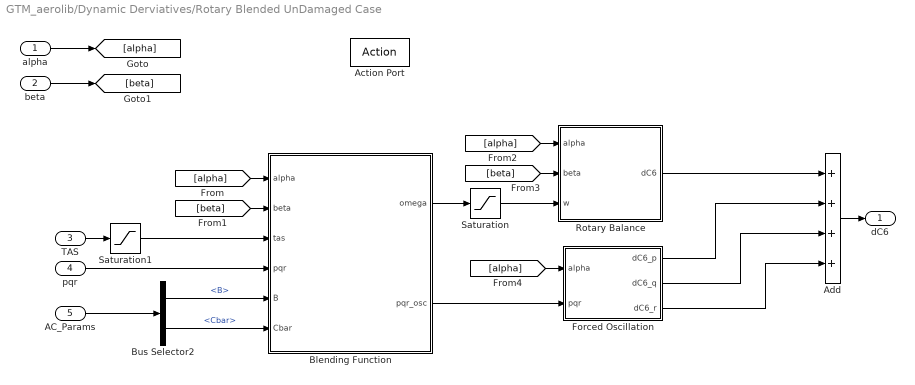
== system GTM_aerolib/Dynamic Derviatives/Rotary Blended UnDamaged Case ==
  alpha : Inport
  beta : Inport  Port=2
  TAS : Inport  Port=3
  pqr : Inport  Port=4
  AC_Params : Inport  Port=5
  Action Port : ActionPort
  Add : Sum  Inputs=++++
  Blending Function : MATLAB Function  TreatAsAtomicUnit=on
  Bus Selector2 : BusSelector  OutputSignals=B,Cbar
  Forced Oscillation : Subsystem
  Rotary Balance : Subsystem
  Saturation : Saturate
  Saturation1 : Saturate  UpperLimit=10000  LowerLimit=1
  dC6 : Outport
  wires:
  Blending Function/1(omega) -> Saturation/1
  Blending Function/2(pqr_osc) -> Forced Oscillation/2(pqr)
  Bus Selector2/1 -> Blending Function/5(B)  "<B>"
  TAS/1 -> Saturation1/1
  AC_Params/1 -> Bus Selector2/1
  [alpha] -> Blending Function/1(alpha)
  alpha/1 -> [alpha]
  beta/1 -> [beta]
  [beta] -> Blending Function/2(beta)
  [alpha] -> Rotary Balance/1(alpha)
  [beta] -> Rotary Balance/2(beta)
  [alpha] -> Forced Oscillation/1(alpha)
  Saturation/1 -> Rotary Balance/3(w)
  Saturation1/1 -> Blending Function/3(tas)
  pqr/1 -> Blending Function/4(pqr)
  Bus Selector2/2 -> Blending Function/6(Cbar)  "<Cbar>"
  Add/1 -> dC6/1
  Rotary Balance/1(dC6) -> Add/1
  Forced Oscillation/1(dC6_p) -> Add/2
  Forced Oscillation/2(dC6_q) -> Add/3
  Forced Oscillation/3(dC6_r) -> Add/4

== system GTM_aerolib/Merged Control Surfaces/Ailerons ==
  alpha : Inport
  beta : Inport  Port=2
  Left : Inport  Port=3
  Right : Inport  Port=4
  Constant1 : Constant  Value=[0:5]  OutDataTypeStr=uint32
  Constant2 : Constant  Value=[0:5]  OutDataTypeStr=uint32
  Gain2 : Gain  Gain=-1
  Negate Lateral : Gain  Gain=[1 -1 1 -1 1 -1]
  PreLookup Index Search : simulink_need_slupdate/PreLookup Index Search  bpData=Aero.dC6_ail.alpha  searchMode=Binary Search  cacheBpFlag=on  outputFlag=off  IndexDataType=uint32  extrapMode=Linear Extrapolation  rangeErrorMode=None
  PreLookup Index Search1 : simulink_need_slupdate/PreLookup Index Search  bpData=Aero.dC6_ail.beta  searchMode=Binary Search  cacheBpFlag=on  outputFlag=off  IndexDataType=uint32  extrapMode=Linear Extrapolation  rangeErrorMode=None
  PreLookup Index Search2 : simulink_need_slupdate/PreLookup Index Search  bpData=Aero.dC6_ail.ail  searchMode=Binary Search  cacheBpFlag=on  outputFlag=off  IndexDataType=uint32  extrapMode=Linear Extrapolation  rangeErrorMode=None
  PreLookup Index Search3 : simulink_need_slupdate/PreLookup Index Search  bpData=Aero.dC6_ail.beta  searchMode=Binary Search  cacheBpFlag=on  outputFlag=off  IndexDataType=uint32  extrapMode=Linear Extrapolation  rangeErrorMode=None
  PreLookup Index Search4 : simulink_need_slupdate/PreLookup Index Search  bpData=Aero.dC6_ail.ail  searchMode=Binary Search  cacheBpFlag=on  outputFlag=off  IndexDataType=uint32  extrapMode=Linear Extrapolation  rangeErrorMode=None
  Sum : Sum  Inputs=+|+
  TableLookup : simulink_need_slupdate/Interpolation (n-D) using PreLookup  numDimsPopupSelect=4  explicitNumDims=2  table=Aero.dC6_ail.data  interpMethod=Linear  extrapMethod=Linear  rangeErrorMode=None  NumSelectionDims=1
  TableLookup1 : simulink_need_slupdate/Interpolation (n-D) using PreLookup  numDimsPopupSelect=4  explicitNumDims=2  table=Aero.dC6_ail.data  interpMethod=Linear  extrapMethod=Linear  rangeErrorMode=None  NumSelectionDims=1
  dC6 : Outport
  wires:
  Left/1 -> PreLookup Index Search2/1
  alpha/1 -> PreLookup Index Search/1
  beta/1 -> Gain2/1, PreLookup Index Search3/1
  Sum/1 -> dC6/1
  PreLookup Index Search/1 -> TableLookup/1, TableLookup1/1
  PreLookup Index Search1/1 -> TableLookup/2
  PreLookup Index Search2/1 -> TableLookup/3
  PreLookup Index Search3/1 -> TableLookup1/2
  Right/1 -> PreLookup Index Search4/1
  PreLookup Index Search4/1 -> TableLookup1/3
  TableLookup/1 -> Negate Lateral/1
  TableLookup1/1 -> Sum/2
  Constant2/1 -> TableLookup/4
  Constant1/1 -> TableLookup1/4
  Negate Lateral/1 -> Sum/1
  Gain2/1 -> PreLookup Index Search1/1

== system GTM_aerolib/Merged Control Surfaces/Elevator//Stab ==
  alpha : Inport
  beta : Inport  Port=2
  stab : Inport  Port=3
  elev : Inport  Port=4
  Assignment to Longitudinal : Assignment  IndexMode=Zero-based  IndexOptions=Index vector (dialog)  Indices=[0 2 4]  OutputSizes=[1 1]
  Constant : Constant  Value=zeros(6,1)
  Constant2 : Constant  Value=[0:2]  OutDataTypeStr=uint32
  PreLookup Index Search : simulink_need_slupdate/PreLookup Index Search  bpData=Aero.dC3_ele.alpha  searchMode=Binary Search  cacheBpFlag=off  outputFlag=off  IndexDataType=uint32  extrapMode=Linear Extrapolation  rangeErrorMode=None
  PreLookup Index Search1 : simulink_need_slupdate/PreLookup Index Search  bpData=Aero.dC3_ele.beta  searchMode=Binary Search  cacheBpFlag=off  outputFlag=off  IndexDataType=uint32  extrapMode=Linear Extrapolation  rangeErrorMode=None
  PreLookup Index Search2 : simulink_need_slupdate/PreLookup Index Search  bpData=Aero.dC3_ele.stab  searchMode=Binary Search  cacheBpFlag=off  outputFlag=off  IndexDataType=uint32  extrapMode=Linear Extrapolation  rangeErrorMode=None
  PreLookup Index Search3 : simulink_need_slupdate/PreLookup Index Search  bpData=Aero.dC3_ele.elev  searchMode=Binary Search  cacheBpFlag=off  outputFlag=off  IndexDataType=uint32  extrapMode=Linear Extrapolation  rangeErrorMode=None
  TableLookup : simulink_need_slupdate/Interpolation (n-D) using PreLookup  numDimsPopupSelect=More...  explicitNumDims=5  table=Aero.dC3_ele.data  interpMethod=Linear  extrapMethod=Linear  rangeErrorMode=None  NumSelectionDims=1
  dC6 : Outport
  wires:
  alpha/1 -> PreLookup Index Search/1
  PreLookup Index Search1/1 -> TableLookup/2
  beta/1 -> PreLookup Index Search1/1
  PreLookup Index Search/1 -> TableLookup/1
  PreLookup Index Search2/1 -> TableLookup/3
  stab/1 -> PreLookup Index Search2/1
  PreLookup Index Search3/1 -> TableLookup/4
  elev/1 -> PreLookup Index Search3/1
  Constant/1 -> Assignment to Longitudinal/1
  TableLookup/1 -> Assignment to Longitudinal/2
  Assignment to Longitudinal/1 -> dC6/1
  Constant2/1 -> TableLookup/5

== system GTM_aerolib/Merged Control Surfaces/ErrorCheck_on_SplitSurface ==
  In1 : Inport
  Abs : Abs  SaturateOnIntegerOverflow=off
  Bus Selector1 : BusSelector  OutputSignals=ELLOB,ELLIB,ELROB,ELRIB,AILL,AILR,RUDU,RUDL,SPLLIB,SPLLOB,SPLRIB,SPLROB,FLAPLI,FLAPLO,FLAPRI,FLAPRO  OutputAsBus=on
  Bus to Vector : BusToVector
  Constant : Constant  Value=1e-4
  Demux : Demux  Outputs=[4 2 2 4 4]
  Gain : Gain  Gain=[1 -1 0 0; 1 0 -1 0; 1 0 0 -1]  Multiplication=Matrix(K*u)
  Gain1 : Gain  Gain=[1 -1 0 0; 1 0 -1 0; 1 0 0 -1]  Multiplication=Matrix(K*u)
  Gain2 : Gain  Gain=[1 -1 0 0; 1 0 -1 0; 1 0 0 -1]  Multiplication=Matrix(K*u)
  Gain3 : Gain  Gain=[1 -1]  Multiplication=Matrix(K*u)
  Gain4 : Gain  Gain=[1 -1]  Multiplication=Matrix(K*u)
  MinMax : MinMax  Function=max
  Mux : Mux  Inputs=5
  Relational Operator : RelationalOperator  Operator=<=  OutDataTypeStr=boolean  InputSameDT=off
  wires:
  Constant/1 -> Relational Operator/2
  Relational Operator/1 -> ?
  MinMax/1 -> Relational Operator/1
  Abs/1 -> MinMax/1
  Mux/1 -> Abs/1
  Gain2/1 -> Mux/5
  Gain1/1 -> Mux/4
  Gain4/1 -> Mux/3
  Gain3/1 -> Mux/2
  Gain/1 -> Mux/1
  Demux/5 -> Gain2/1
  Demux/3 -> Gain4/1
  Demux/2 -> Gain3/1
  Demux/4 -> Gain1/1
  Demux/1 -> Gain/1
  Bus to Vector/1 -> Demux/1
  Bus Selector1/1 -> Bus to Vector/1
  In1/1 -> Bus Selector1/1

== system GTM_aerolib/Merged Control Surfaces/Flap ==
  alpha : Inport
  flap : Inport  Port=2
  Assignment to Longitudinal : Assignment  IndexMode=Zero-based  IndexOptions=Index vector (dialog)  Indices=[0 2 4]  OutputSizes=[1 1]
  Constant : Constant  Value=zeros(6,1)
  Constant2 : Constant  Value=[0:2]  OutDataTypeStr=uint32
  PreLookup Index Search : simulink_need_slupdate/PreLookup Index Search  bpData=Aero.dC3_flp.flap  searchMode=Binary Search  cacheBpFlag=on  outputFlag=off  IndexDataType=uint32  extrapMode=Linear Extrapolation  rangeErrorMode=None
  PreLookup Index Search1 : simulink_need_slupdate/PreLookup Index Search  bpData=Aero.dC3_flp.alpha  searchMode=Binary Search  cacheBpFlag=on  outputFlag=off  IndexDataType=uint32  extrapMode=Linear Extrapolation  rangeErrorMode=None
  TableLookup : simulink_need_slupdate/Interpolation (n-D) using PreLookup  numDimsPopupSelect=3  explicitNumDims=2  table=Aero.dC3_flp.data  interpMethod=Linear  extrapMethod=Linear  rangeErrorMode=None  NumSelectionDims=1
  dC6 : Outport
  wires:
  flap/1 -> PreLookup Index Search/1
  PreLookup Index Search/1 -> TableLookup/2
  alpha/1 -> PreLookup Index Search1/1
  PreLookup Index Search1/1 -> TableLookup/1
  Constant2/1 -> TableLookup/3
  Constant/1 -> Assignment to Longitudinal/1
  TableLookup/1 -> Assignment to Longitudinal/2
  Assignment to Longitudinal/1 -> dC6/1

== system GTM_aerolib/Merged Control Surfaces/Gear ==
  alpha : Inport
  gear : Inport  Port=2
  Assignment to Longitudinal : Assignment  IndexMode=Zero-based  IndexOptions=Index vector (dialog)  Indices=[0 2 4]  OutputSizes=[1 1]
  Compare To Zero : simulink/Logic and Bit Operations/Compare To Zero  SystemSampleTime=-1  relop=~=  LogicOutDataTypeMode=uint8  ZeroCross=off
  Constant : Constant  Value=zeros(6,1)
  Constant2 : Constant  Value=[0:2]  OutDataTypeStr=uint32
  Data Type Conversion2 : DataTypeConversion  OutDataTypeStr=uint32  SaturateOnIntegerOverflow=off  RndMeth=Floor
  PreLookup Index Search1 : simulink_need_slupdate/PreLookup Index Search  bpData=Aero.dC3_lgr.alpha  searchMode=Binary Search  cacheBpFlag=on  outputFlag=off  IndexDataType=uint32  extrapMode=Linear Extrapolation  rangeErrorMode=None
  TableLookup : simulink_need_slupdate/Interpolation (n-D) using PreLookup  numDimsPopupSelect=3  explicitNumDims=2  table=Aero.dC3_lgr.data  interpMethod=Linear  extrapMethod=Linear  rangeErrorMode=None  NumSelectionDims=2
  dC6 : Outport
  wires:
  gear/1 -> Compare To Zero/1
  Compare To Zero/1 -> Data Type Conversion2/1
  alpha/1 -> PreLookup Index Search1/1
  PreLookup Index Search1/1 -> TableLookup/1
  Constant2/1 -> TableLookup/3
  TableLookup/1 -> Assignment to Longitudinal/2
  Constant/1 -> Assignment to Longitudinal/1
  Assignment to Longitudinal/1 -> dC6/1
  Data Type Conversion2/1 -> TableLookup/2

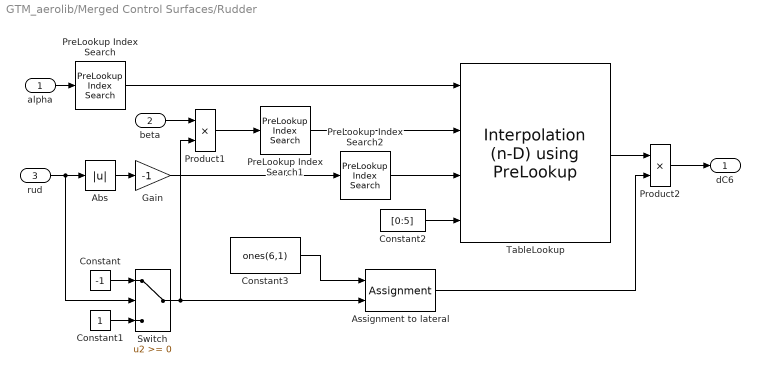
== system GTM_aerolib/Merged Control Surfaces/Rudder ==
  alpha : Inport
  beta : Inport  Port=2
  rud : Inport  Port=3
  Abs : Abs  SaturateOnIntegerOverflow=off
  Assignment to lateral : Assignment  IndexMode=Zero-based  IndexOptions=Index vector (dialog)  Indices=[1 3 5]  OutputSizes=[1 1]
  Constant : Constant  Value=-1
  Constant1 : Constant
  Constant2 : Constant  Value=[0:5]  OutDataTypeStr=uint32
  Constant3 : Constant  Value=ones(6,1)
  Gain : Gain  Gain=-1
  PreLookup Index Search : simulink_need_slupdate/PreLookup Index Search  bpData=Aero.dC6_rud.alpha  searchMode=Binary Search  cacheBpFlag=on  outputFlag=off  IndexDataType=uint32  extrapMode=Linear Extrapolation  rangeErrorMode=None
  PreLookup Index Search1 : simulink_need_slupdate/PreLookup Index Search  bpData=Aero.dC6_rud.beta  searchMode=Binary Search  cacheBpFlag=on  outputFlag=off  IndexDataType=uint32  extrapMode=Linear Extrapolation  rangeErrorMode=None
  PreLookup Index Search2 : simulink_need_slupdate/PreLookup Index Search  bpData=Aero.dC6_rud.rud  searchMode=Binary Search  cacheBpFlag=on  outputFlag=off  IndexDataType=uint32  extrapMode=Linear Extrapolation  rangeErrorMode=None
  Product1 : Product  RndMeth=Zero
  Product2 : Product  RndMeth=Zero
  Switch : Switch  SaturateOnIntegerOverflow=off  InputSameDT=off
  TableLookup : simulink_need_slupdate/Interpolation (n-D) using PreLookup  numDimsPopupSelect=4  explicitNumDims=2  table=Aero.dC6_rud.data  interpMethod=Linear  extrapMethod=Linear  rangeErrorMode=None  NumSelectionDims=1
  dC6 : Outport
  wires:
  rud/1 -> Abs/1, Switch/2
  Abs/1 -> Gain/1
  Gain/1 -> PreLookup Index Search2/1
  Product1/1 -> PreLookup Index Search1/1
  alpha/1 -> PreLookup Index Search/1
  beta/1 -> Product1/1
  Product2/1 -> dC6/1
  Constant/1 -> Switch/1
  Constant1/1 -> Switch/3
  Switch/1 -> Product1/2, Assignment to lateral/2
  Constant3/1 -> Assignment to lateral/1
  PreLookup Index Search/1 -> TableLookup/1
  PreLookup Index Search1/1 -> TableLookup/2
  PreLookup Index Search2/1 -> TableLookup/3
  Assignment to lateral/1 -> Product2/2
  TableLookup/1 -> Product2/1
  Constant2/1 -> TableLookup/4

== system GTM_aerolib/Merged Control Surfaces/Spoilers ==
  alpha : Inport
  beta : Inport  Port=2
  Left : Inport  Port=3
  Right : Inport  Port=4
  Constant1 : Constant  Value=[0:5]  OutDataTypeStr=uint32
  Constant2 : Constant  Value=[0:5]  OutDataTypeStr=uint32
  Gain2 : Gain  Gain=-1
  Negate Lateral : Gain  Gain=[1 -1 1 -1 1 -1]
  PreLookup Index Search : simulink_need_slupdate/PreLookup Index Search  bpData=Aero.dC6_spo.alpha  searchMode=Binary Search  cacheBpFlag=on  outputFlag=off  IndexDataType=uint32  extrapMode=Linear Extrapolation  rangeErrorMode=None
  PreLookup Index Search1 : simulink_need_slupdate/PreLookup Index Search  bpData=Aero.dC6_spo.beta  searchMode=Binary Search  cacheBpFlag=on  outputFlag=off  IndexDataType=uint32  extrapMode=Linear Extrapolation  rangeErrorMode=None
  PreLookup Index Search2 : simulink_need_slupdate/PreLookup Index Search  bpData=Aero.dC6_spo.spo  searchMode=Binary Search  cacheBpFlag=on  outputFlag=off  IndexDataType=uint32  extrapMode=Linear Extrapolation  rangeErrorMode=None
  PreLookup Index Search3 : simulink_need_slupdate/PreLookup Index Search  bpData=Aero.dC6_spo.beta  searchMode=Binary Search  cacheBpFlag=on  outputFlag=off  IndexDataType=uint32  extrapMode=Linear Extrapolation  rangeErrorMode=None
  PreLookup Index Search4 : simulink_need_slupdate/PreLookup Index Search  bpData=Aero.dC6_spo.spo  searchMode=Binary Search  cacheBpFlag=on  outputFlag=off  IndexDataType=uint32  extrapMode=Linear Extrapolation  rangeErrorMode=None
  Sum : Sum  Inputs=+|+
  TableLookup : simulink_need_slupdate/Interpolation (n-D) using PreLookup  numDimsPopupSelect=4  explicitNumDims=2  table=Aero.dC6_spo.data  interpMethod=Linear  extrapMethod=Linear  rangeErrorMode=None  NumSelectionDims=1
  TableLookup1 : simulink_need_slupdate/Interpolation (n-D) using PreLookup  numDimsPopupSelect=4  explicitNumDims=2  table=Aero.dC6_spo.data  interpMethod=Linear  extrapMethod=Linear  rangeErrorMode=None  NumSelectionDims=1
  dC6 : Outport
  wires:
  Left/1 -> PreLookup Index Search2/1
  alpha/1 -> PreLookup Index Search/1
  beta/1 -> PreLookup Index Search3/1, Gain2/1
  Sum/1 -> dC6/1
  PreLookup Index Search/1 -> TableLookup/1, TableLookup1/1
  PreLookup Index Search1/1 -> TableLookup/2
  PreLookup Index Search2/1 -> TableLookup/3
  PreLookup Index Search3/1 -> TableLookup1/2
  TableLookup1/1 -> Sum/2
  TableLookup/1 -> Negate Lateral/1
  Right/1 -> PreLookup Index Search4/1
  PreLookup Index Search4/1 -> TableLookup1/3
  Constant2/1 -> TableLookup/4
  Constant1/1 -> TableLookup1/4
  Gain2/1 -> PreLookup Index Search1/1
  Negate Lateral/1 -> Sum/1

== system GTM_aerolib/Basic Airframe/DamageEffects/Switch Case Action Subsystem ==
  alpha : Inport
  beta : Inport  Port=2
  damage_case : Inport  Port=3
  Action Port : ActionPort  ActionPortLabel=case: { }
  AlphaLookup : PreLookup  BreakpointsData=Aero.dC6_damage.bas.alpha  BeginIndexSearchUsingPreviousIndexResult=on  ExtrapMethod=Linear
  BetaLookup : PreLookup  BreakpointsData=Aero.dC6_damage.bas.beta  ExtrapMethod=Linear
  Constant : Constant  Value=uint32(1)
  Constant4 : Constant  Value=[0:5]  OutDataTypeStr=uint32
  Interpolation Using Prelookup : Interpolation_n-D  NumberOfTableDimensions=4  Table=Aero.dC6_damage.bas.data  ExtrapMethod=Clip  NumSelectionDims=2
      settings: InputPortMap=u0,u1,u2,u3,u4,u5
  Subtract : Sum  Inputs=+-
  dC6_dam : Outport  InitialOutput=zeros(6,1)
  wires:
  Constant4/1 -> Interpolation Using Prelookup/6
  alpha/1 -> AlphaLookup/1
  beta/1 -> BetaLookup/1
  Interpolation Using Prelookup/1 -> dC6_dam/1
  AlphaLookup/1 -> Interpolation Using Prelookup/1
  AlphaLookup/2 -> Interpolation Using Prelookup/2
  BetaLookup/1 -> Interpolation Using Prelookup/3
  BetaLookup/2 -> Interpolation Using Prelookup/4
  damage_case/1 -> Subtract/1
  Subtract/1 -> Interpolation Using Prelookup/5
  Constant/1 -> Subtract/2

== system GTM_aerolib/Basic Airframe/DamageEffects/Switch Case Action Subsystem2 ==
  Action Port : ActionPort  ActionPortLabel=default: { }
  Constant4 : Constant  Value=zeros(6,1)  OutDataTypeStr=double
  Zeros : Outport  InitialOutput=zeros(6,1)
  wires:
  Constant4/1 -> Zeros/1

== system GTM_aerolib/Control Surfaces/Elevator//Stab1/Stab//Elev Table ==
  alpha_k : Inport
  alpha_f : Inport  Port=2
  beta_k : Inport  Port=3
  beta_f : Inport  Port=4
  stab_k : Inport  Port=5
  stab_f : Inport  Port=6
  elev : Inport  Port=7
  Assignment to Longitudinal : Assignment  IndexMode=Zero-based  IndexOptions=Index vector (dialog)  Indices=[0 2 4]  OutputSizes=[1 1]
  Constant : Constant  Value=zeros(6,1)
  Constant2 : Constant  Value=[0:2]  OutDataTypeStr=uint32
  Interpolation Using Prelookup : Interpolation_n-D  NumberOfTableDimensions=5  Table=Aero.dC3_ele.data  NumSelectionDims=1
      settings: InputPortMap=u0,u1,u2,u3,u4,u5,u6,u7,u8
  Prelookup4 : PreLookup  BreakpointsData=Aero.dC3_ele.elev  IndexSearchMethod=Linear search  BeginIndexSearchUsingPreviousIndexResult=on  ExtrapMethod=Linear
  dC6 : Outport
  wires:
  Assignment to Longitudinal/1 -> dC6/1
  Interpolation Using Prelookup/1 -> Assignment to Longitudinal/2
  Constant/1 -> Assignment to Longitudinal/1
  elev/1 -> Prelookup4/1
  stab_k/1 -> Interpolation Using Prelookup/5
  beta_k/1 -> Interpolation Using Prelookup/3
  alpha_k/1 -> Interpolation Using Prelookup/1
  alpha_f/1 -> Interpolation Using Prelookup/2
  beta_f/1 -> Interpolation Using Prelookup/4
  stab_f/1 -> Interpolation Using Prelookup/6
  Prelookup4/1 -> Interpolation Using Prelookup/7
  Prelookup4/2 -> Interpolation Using Prelookup/8
  Constant2/1 -> Interpolation Using Prelookup/9

== system GTM_aerolib/Control Surfaces/Elevator//Stab1/Stab//Elev Table0 ==
  alpha_k : Inport
  alpha_f : Inport  Port=2
  beta_k : Inport  Port=3
  beta_f : Inport  Port=4
  stab_k : Inport  Port=5
  stab_f : Inport  Port=6
  elev : Inport  Port=7
  Assignment to Longitudinal : Assignment  IndexMode=Zero-based  IndexOptions=Index vector (dialog)  Indices=[0 2 4]  OutputSizes=[1 1]
  Constant : Constant  Value=zeros(6,1)
  Constant2 : Constant  Value=[0:2]  OutDataTypeStr=uint32
  Interpolation Using Prelookup : Interpolation_n-D  NumberOfTableDimensions=5  Table=Aero.dC3_ele.data  NumSelectionDims=1
      settings: InputPortMap=u0,u1,u2,u3,u4,u5,u6,u7,u8
  Prelookup4 : PreLookup  BreakpointsData=Aero.dC3_ele.elev  IndexSearchMethod=Linear search  BeginIndexSearchUsingPreviousIndexResult=on  ExtrapMethod=Linear
  dC6 : Outport
  wires:
  Assignment to Longitudinal/1 -> dC6/1
  Interpolation Using Prelookup/1 -> Assignment to Longitudinal/2
  Constant/1 -> Assignment to Longitudinal/1
  elev/1 -> Prelookup4/1
  stab_k/1 -> Interpolation Using Prelookup/5
  beta_k/1 -> Interpolation Using Prelookup/3
  alpha_k/1 -> Interpolation Using Prelookup/1
  alpha_f/1 -> Interpolation Using Prelookup/2
  beta_f/1 -> Interpolation Using Prelookup/4
  stab_f/1 -> Interpolation Using Prelookup/6
  Prelookup4/1 -> Interpolation Using Prelookup/7
  Prelookup4/2 -> Interpolation Using Prelookup/8
  Constant2/1 -> Interpolation Using Prelookup/9

== system GTM_aerolib/Control Surfaces/Elevator//Stab1/Stab//Elev Table1 ==
  alpha_k : Inport
  alpha_f : Inport  Port=2
  beta_k : Inport  Port=3
  beta_f : Inport  Port=4
  stab_k : Inport  Port=5
  stab_f : Inport  Port=6
  elev : Inport  Port=7
  Assignment to Longitudinal : Assignment  IndexMode=Zero-based  IndexOptions=Index vector (dialog)  Indices=[0 2 4]  OutputSizes=[1 1]
  Constant : Constant  Value=zeros(6,1)
  Constant2 : Constant  Value=[0:2]  OutDataTypeStr=uint32
  Interpolation Using Prelookup : Interpolation_n-D  NumberOfTableDimensions=5  Table=Aero.dC3_ele.data  NumSelectionDims=1
      settings: InputPortMap=u0,u1,u2,u3,u4,u5,u6,u7,u8
  Prelookup4 : PreLookup  BreakpointsData=Aero.dC3_ele.elev  IndexSearchMethod=Linear search  BeginIndexSearchUsingPreviousIndexResult=on  ExtrapMethod=Linear
  dC6 : Outport
  wires:
  Assignment to Longitudinal/1 -> dC6/1
  Interpolation Using Prelookup/1 -> Assignment to Longitudinal/2
  Constant/1 -> Assignment to Longitudinal/1
  elev/1 -> Prelookup4/1
  stab_k/1 -> Interpolation Using Prelookup/5
  beta_k/1 -> Interpolation Using Prelookup/3
  alpha_k/1 -> Interpolation Using Prelookup/1
  alpha_f/1 -> Interpolation Using Prelookup/2
  beta_f/1 -> Interpolation Using Prelookup/4
  stab_f/1 -> Interpolation Using Prelookup/6
  Prelookup4/1 -> Interpolation Using Prelookup/7
  Prelookup4/2 -> Interpolation Using Prelookup/8
  Constant2/1 -> Interpolation Using Prelookup/9
